simulink model "analog_ext"  (Simulink 7.6)
settings: Solver=FixedStepDiscrete  StartTime=0.0  StopTime=10000  FixedStep=1  RelTol=1e-3
libraries: simulink x12
settings Model: Creator=jordan  LastModifiedBy=jordan
settings DataIOCC: LimitDataPoints=off  SaveOutput=off  SignalLogging=off  DSMLogging=off  SaveTime=off
settings OptimizationCC: BlockReduction=off  ConditionallyExecuteInputs=off

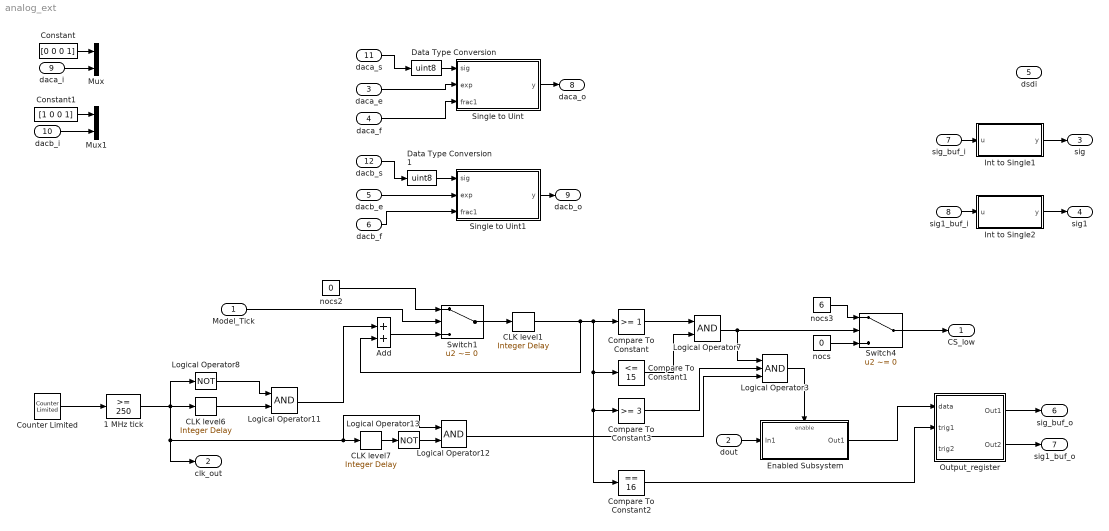
== system analog_ext ==
  Model_Tick : Inport  OutDataTypeStr=boolean
  dout : Inport  Port=2  OutDataTypeStr=boolean
  daca_e : Inport  Port=3  OutDataTypeStr=uint8
  daca_f : Inport  Port=4  OutDataTypeStr=fixdt(0,24,0)
  dacb_e : Inport  Port=5  OutDataTypeStr=uint8
  dacb_f : Inport  Port=6  OutDataTypeStr=fixdt(0,24,0)
  sig_buf_i : Inport  Port=7  OutDataTypeStr=fixdt(0,12,0)
  sig1_buf_i : Inport  Port=8  OutDataTypeStr=fixdt(0,12,0)
  daca_i : Inport  Port=9  OutDataTypeStr=boolean  PortDimensions=12
  dacb_i : Inport  Port=10  OutDataTypeStr=boolean  PortDimensions=12
  daca_s : Inport  Port=11  OutDataTypeStr=boolean
  dacb_s : Inport  Port=12  OutDataTypeStr=boolean
  1 MHz tick : simulink/Logic and Bit Operations/Compare To Constant  SystemSampleTime=-1  relop=>=  const=250  LogicOutDataTypeMode=boolean
  Add : Sum  OutDataTypeStr=fixdt(0,7,0)  SaturateOnIntegerOverflow=on
  CLK level1 : simulink/Discrete/Integer Delay  NumDelays=1  vinit=0.0  samptime=-1
  CLK level6 : simulink/Discrete/Integer Delay  NumDelays=1  vinit=0.0  samptime=-1
  CLK level7 : simulink/Discrete/Integer Delay  NumDelays=1  vinit=0.0  samptime=-1
  Compare To Constant : simulink/Logic and Bit Operations/Compare To Constant  SystemSampleTime=-1  relop=>=  const=1  LogicOutDataTypeMode=boolean
  Compare To Constant1 : simulink/Logic and Bit Operations/Compare To Constant  SystemSampleTime=-1  relop=<=  const=15  LogicOutDataTypeMode=boolean
  Compare To Constant2 : simulink/Logic and Bit Operations/Compare To Constant  SystemSampleTime=-1  relop===  const=16  LogicOutDataTypeMode=boolean
  Compare To Constant3 : simulink/Logic and Bit Operations/Compare To Constant  SystemSampleTime=-1  relop=>=  const=3  LogicOutDataTypeMode=boolean
  Constant : Constant  Value=[0 0 0 1]  OutDataTypeStr=boolean
  Constant1 : Constant  Value=[1 0 0 1]  OutDataTypeStr=boolean
  Counter Limited : simulink/Sources/Counter Limited  SystemSampleTime=-1  uplimit=500  tsamp=-1
  Data Type Conversion : DataTypeConversion  OutDataTypeStr=uint8
  Data Type Conversion1 : DataTypeConversion  OutDataTypeStr=uint8
  Enabled Subsystem : Subsystem  TreatAsAtomicUnit=on
  Int to Single1 : Stateflow chart  TreatAsAtomicUnit=on
  Int to Single2 : Stateflow chart  TreatAsAtomicUnit=on
  Logical Operator11 : Logic  AllPortsSameDT=off  OutDataTypeStr=boolean
  Logical Operator12 : Logic  AllPortsSameDT=off  OutDataTypeStr=boolean
  Logical Operator13 : Logic  Operator=NOT  AllPortsSameDT=off  OutDataTypeStr=boolean
  Logical Operator3 : Logic  Inputs=3  AllPortsSameDT=off  OutDataTypeStr=boolean
  Logical Operator7 : Logic  AllPortsSameDT=off  OutDataTypeStr=boolean
  Logical Operator8 : Logic  Operator=NOT  AllPortsSameDT=off  OutDataTypeStr=boolean
  Mux : Mux  Inputs=2
  Mux1 : Mux  Inputs=2
  Output_register : Subsystem
  Single to Uint : Stateflow chart  TreatAsAtomicUnit=on
  Single to Uint1 : Stateflow chart  TreatAsAtomicUnit=on
  Switch1 : Switch  Criteria=u2 ~= 0
  Switch4 : Switch  Criteria=u2 ~= 0
  nocs : Constant  Value=0  OutDataTypeStr=fixdt(0,3,0)
  nocs2 : Constant  Value=0  OutDataTypeStr=fixdt(0,7,0)
  nocs3 : Constant  Value=6  OutDataTypeStr=fixdt(0,3,0)
  CS_low : Outport  OutDataTypeStr=fixdt(0,3,0)
  clk_out : Outport  Port=2  OutDataTypeStr=boolean
  sig : Outport  Port=3  OutDataTypeStr=uint32  PortDimensions=1
  sig1 : Outport  Port=4  OutDataTypeStr=uint32  PortDimensions=1
  dsdi : Outport  Port=5  OutDataTypeStr=boolean
  sig_buf_o : Outport  Port=6  OutDataTypeStr=boolean  PortDimensions=12
  sig1_buf_o : Outport  Port=7  OutDataTypeStr=boolean  PortDimensions=12
  daca_o : Outport  Port=8  OutDataTypeStr=fixdt(0,12,0)
  dacb_o : Outport  Port=9  OutDataTypeStr=fixdt(0,12,0)
  wires:
  Counter Limited/1 -> 1 MHz tick/1
  Constant/1 -> Mux/1
  Constant1/1 -> Mux1/1
  Output_register/1(Out1) -> sig_buf_o/1
  Output_register/2(Out2) -> sig1_buf_o/1
  Int to Single1/1(y) -> sig/1
  Int to Single2/1(y) -> sig1/1
  Single to Uint/1(y) -> daca_o/1
  Single to Uint1/1(y) -> dacb_o/1
  daca_s/1 -> Data Type Conversion/1
  daca_e/1 -> Single to Uint/2(exp)
  daca_f/1 -> Single to Uint/3(frac1)
  dacb_e/1 -> Single to Uint1/2(exp)
  dacb_f/1 -> Single to Uint1/3(frac1)
  sig_buf_i/1 -> Int to Single1/1(u)
  sig1_buf_i/1 -> Int to Single2/1(u)
  daca_i/1 -> Mux/2
  dacb_i/1 -> Mux1/2
  dacb_s/1 -> Data Type Conversion1/1
  Data Type Conversion/1 -> Single to Uint/1(sig)
  Data Type Conversion1/1 -> Single to Uint1/1(sig)
  dout/1 -> Enabled Subsystem/1(In1)
  Add/1 -> Switch1/3
  CLK level1/1 -> Add/2, Compare To Constant/1, Compare To Constant1/1, Compare To Constant3/1, Compare To Constant2/1
  Logical Operator11/1 -> Add/1
  Switch1/1 -> CLK level1/1
  Model_Tick/1 -> Switch1/2
  nocs2/1 -> Switch1/1
  Compare To Constant/1 -> Logical Operator7/1
  Compare To Constant1/1 -> Logical Operator7/2
  Logical Operator7/1 -> Switch4/2, Logical Operator3/1
  Switch4/1 -> CS_low/1
  nocs3/1 -> Switch4/1
  Compare To Constant3/1 -> Logical Operator3/2
  Logical Operator3/1 -> Enabled Subsystem/Enable
  nocs/1 -> Switch4/3
  CLK level6/1 -> Logical Operator11/2
  1 MHz tick/1 -> CLK level6/1, Logical Operator8/1, clk_out/1, CLK level7/1, Logical Operator12/1
  Logical Operator8/1 -> Logical Operator11/1
  CLK level7/1 -> Logical Operator13/1
  Logical Operator13/1 -> Logical Operator12/2
  Logical Operator12/1 -> Logical Operator3/3
  Enabled Subsystem/1(Out1) -> Output_register/1(data)
  Compare To Constant2/1 -> Output_register/2(trig1)

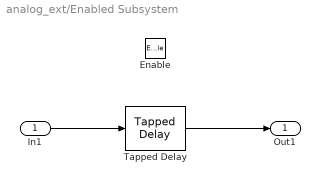
== system analog_ext/Enabled Subsystem ==
  In1 : Inport
  Enable : EnablePort
  Tapped Delay : simulink/Discrete/Tapped Delay  vinit=0.0  samptime=-1  NumDelays=12  DelayOrder=Oldest  includeCurrent=off
  Out1 : Outport  InitialOutput=0
  wires:
  In1/1 -> Tapped Delay/1
  Tapped Delay/1 -> Out1/1

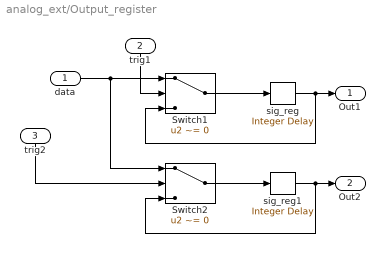
== system analog_ext/Output_register ==
  data : Inport
  trig1 : Inport  Port=2
  trig2 : Inport  Port=3
  Switch1 : Switch  Criteria=u2 ~= 0
  Switch2 : Switch  Criteria=u2 ~= 0
  sig_reg : simulink/Discrete/Integer Delay  NumDelays=1  vinit=0.0  samptime=-1
  sig_reg1 : simulink/Discrete/Integer Delay  NumDelays=1  vinit=0.0  samptime=-1
  Out1 : Outport
  Out2 : Outport  Port=2
  wires:
  Switch1/1 -> sig_reg/1
  sig_reg/1 -> Switch1/3, Out1/1
  Switch2/1 -> sig_reg1/1
  sig_reg1/1 -> Switch2/3, Out2/1
  trig1/1 -> Switch1/2
  data/1 -> Switch1/1, Switch2/1
  trig2/1 -> Switch2/2

== matlab function Int to Single1 ==
  data: u input fixdt(0,12,0); y output uint32
function y = fcn(u)
%#eml

sig=uint8(0);
exp=uint8(0);
frac=fi(0,0,23,0);

%Transform two's complement integer into unnormalized
%single number
buf=fi(0,0,12,0);
sig=uint8(0);
buf=u;
frac1=fi(buf,0,23,0);

%Normalize floating-point number
buf1=fi(frac1,0,24,0);
p=fi(0,0,5,0);
mask=fi(2^22,0,24,0);
for ind=1:23
    c=bitand(buf1,mask);
    if (c==0)
        buf1=bitshift(buf1,1);
        p=fi(p+1,0,5,0);
    end
end
p=fi(p+1,0,5,0);
buf1=bitshift(fi(frac1,0,24,0),uint8(p));
mask1=fi(2^23-1,0,24,0);
buf1=bitand(buf1,mask1);
frac=fi(buf1,0,23,0);
exp=uint8(127+(22-p));

%Compose floating-point number
z=uint32(0);
if sig
    z=uint32(bitshift(uint32(1),31));
end
buf2=uint32(bitshift(uint32(exp),23));
z=bitor(z,buf2);
z=bitor(z,uint32(frac));
y=z;

== matlab function Int to Single2 ==
  data: u input fixdt(0,12,0); y output uint32
function y = fcn(u)
%#eml

sig=uint8(0);
exp=uint8(0);
frac=fi(0,0,23,0);

%Transform two's complement integer into unnormalized
%single number
buf=fi(0,0,12,0);
sig=uint8(0);
buf=u;
frac1=fi(buf,0,23,0);

%Normalize floating-point number
buf1=fi(frac1,0,24,0);
p=fi(0,0,5,0);
mask=fi(2^22,0,24,0);
for ind=1:23
    c=bitand(buf1,mask);
    if (c==0)
        buf1=bitshift(buf1,1);
        p=fi(p+1,0,5,0);
    end
end
p=fi(p+1,0,5,0);
buf1=bitshift(fi(frac1,0,24,0),uint8(p));
mask1=fi(2^23-1,0,24,0);
buf1=bitand(buf1,mask1);
frac=fi(buf1,0,23,0);
exp=uint8(127+(22-p));

%Compose floating-point number
z=uint32(0);
if sig
    z=uint32(bitshift(uint32(1),31));
end
buf2=uint32(bitshift(uint32(exp),23));
z=bitor(z,buf2);
z=bitor(z,uint32(frac));
y=z;

== matlab function Single to Uint ==
  data: sig input uint8; y output fixdt(0,12,0); exp input uint8; frac1 input fixdt(0,24,0)
function y = fcn(sig, exp, frac1)
%#eml

y=fi(0,0,12,0);
z=int16(0);
if (sig==0)
    if (exp>=127)
        buf=uint32(frac1);
        z=int16(exp)-150;
        y=fi(bitshift(buf,z),0,12,0); %-23+(exp-127)
    end
end

== matlab function Single to Uint1 ==
  data: sig input uint8; y output fixdt(0,12,0); exp input uint8; frac1 input fixdt(0,24,0)
function y = fcn(sig, exp, frac1)
%#eml

y=fi(0,0,12,0);
z=int16(0);
if (sig==0)
    if (exp>=127)
        buf=uint32(frac1);
        z=int16(exp)-150;
        y=fi(bitshift(buf,z),0,12,0); %-23+(exp-127)
    end
end
